simulink model "StemCellStateflow_min"  (R2025b)
settings: Solver=ode4  StartTime=0.0  StopTime=100  FixedStep=0.1  RelTol=1e-3
values from neighbouring files (symbols this model uses):
  RATE_2P = 0.15    [esercizione3_week2.m]
  RATE_2S = 0.30    (= 0.3)    [esercizione3_week2.m]
  RATE_ASYM = 0.50    (= 0.5)    [esercizione3_week2.m]
  RATE_DEATH = 0.05    [esercizione3_week2.m]
  RATE_GRAN = 0.60    (= 0.6)    [esercizione3_week2.m]
  RATE_MACRO = 0.40    (= 0.4)    [esercizione3_week2.m]
settings Model: Creator=aleqs  LastModifiedBy=aleqs

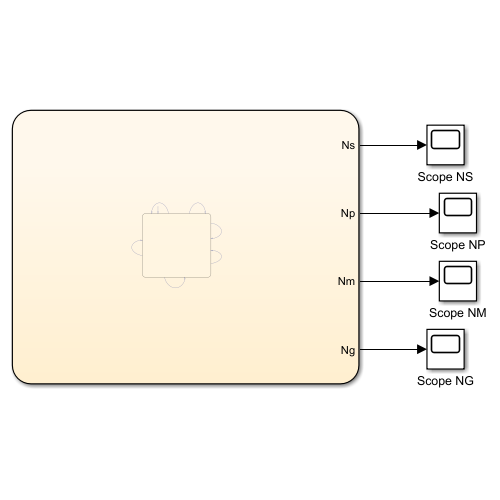
[thumbnail: Simulink's stored preview of the top-level diagram]
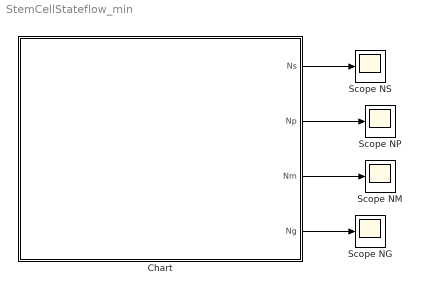
== system StemCellStateflow_min ==
  Chart : Stateflow chart  TreatAsAtomicUnit=on
  Scope NG : Scope
      settings: ActiveDisplayYMinimum=-16.249999999999996  ActiveDisplayYMaximum=146.25  DataLoggingVariableName=ScopeData3
  Scope NM : Scope
      settings: ActiveDisplayYMinimum=-12.630434782608695  ActiveDisplayYMaximum=96.307065217391312  DataLoggingVariableName=ScopeData2
  Scope NP : Scope
      settings: ActiveDisplayYMinimum=35.770917999061176  ActiveDisplayYMaximum=97.75034137796743
  Scope NS : Scope
      settings: ActiveDisplayYMinimum=83.087517832880422  ActiveDisplayYMaximum=137.78529908288044
  wires:
  Chart/4(Ng) -> Scope NG/1
  Chart/3(Nm) -> Scope NM/1
  Chart/2(Np) -> Scope NP/1
  Chart/1(Ns) -> Scope NS/1

== stateflow chart StemCellStateflow_min/Chart ==
  settings: updateMethod=DISCRETE  sampleTime=0.1
  state StemModel
    entry:
    % inizializza orologio
    t = 0;
    % estrai tempi esponenziali per STEM (rate * Ns)
    tau_2S    = -log(rand()) / (RATE_2S  * Ns);
    tau_ASYM  = -log(rand()) / (RATE_ASYM  * Ns);
    tau_2P    = -log(rand()) / (RATE_2P  * Ns);
    tau_DEATH = -log(rand()) / (RATE_DEATH * Ns);
    % estrai tempi per PROGENITORI (se >0)
    if Np > 0
    tau_MACRO = -log(rand()) / (RATE_MACRO * Np);
    tau_GRAN  = -log(rand()) / (RATE_GRAN  * Np);
    else
    tau_MACRO = inf;
    tau_GRAN  = inf;
    end
    during:
    % integra il tempo con passo fisso
    t = t + 0.1;
  StemModel -> StemModel [order 5] : [t >= tau_MACRO && ...
      |  tau_MACRO <= tau_GRAN && tau_MACRO <= tau_2S && ...
      |  tau_MACRO <= tau_ASYM && tau_MACRO <= tau_2P && ...
      |  tau_MACRO <= tau_DEATH && Np > 0]
      | {
      |     Np = Np - 1;
      |     Nm = Nm + 1;
      |     t = 0;
      | }
  StemModel -> StemModel [order 4] : [t >= tau_DEATH && ...
      |  tau_DEATH <= tau_2S && tau_DEATH <= tau_ASYM && tau_DEATH <= tau_2P && ...
      |  tau_DEATH <= tau_MACRO && tau_DEATH <= tau_GRAN && Ns > 0]
      | {
      |     Ns = Ns - 1;
      |     t = 0;
      | }
  (default) -> StemModel
  StemModel -> StemModel [order 6] : [t >= tau_GRAN && tau_GRAN <= tau_MACRO && ...
      |  tau_GRAN <= tau_2S && tau_GRAN <= tau_ASYM && tau_GRAN <= tau_2P && ...
      | tau_GRAN <= tau_DEATH && Np > 0]
      | {
      |     Np = Np - 1;
      |     Ng = Ng + 1;
      |     t = 0;
      | }
  StemModel -> StemModel [order 3] : [t >= tau_2P && ...
      |  tau_2P <= tau_2S && tau_2P <= tau_ASYM && tau_2P <= tau_DEATH && ...
      |  tau_2P <= tau_MACRO && tau_2P <= tau_GRAN && Ns > 0]
      | {
      |     Ns = Ns - 1;
      |     Np = Np + 2;
      |     t = 0;
      | }
  StemModel -> StemModel [order 1] : [t >= tau_2S && ...
      |  tau_2S <= tau_ASYM && tau_2S <= tau_2P && tau_2S <= tau_DEATH && ...
      |  tau_2S <= tau_MACRO && tau_2S <= tau_GRAN && Ns > 0]
      | {
      |     Ns = Ns + 1;
      |     t = 0;
      | }
  StemModel -> StemModel [order 2] : [t >= tau_ASYM && ...
      |  tau_ASYM <= tau_2S && tau_ASYM <= tau_2P && tau_ASYM <= tau_DEATH && ...
      |  tau_ASYM <= tau_MACRO && tau_ASYM <= tau_GRAN && Ns > 0]
      | {
      |     Np = Np + 1;
      |     t = 0;
      | }
  data: Ns output =INITIAL_STEM; t local =0; tau_2S local; tau_ASYM local; Np output =INITIAL_PROG; tau_2P local; tau_DEATH local; Nm output =0; Ng output =0; tau_MACRO local; tau_GRAN local; RATE_2S parameter; RATE_2P parameter; RATE_GRAN parameter; RATE_ASYM parameter; RATE_MACRO parameter; RATE_DEATH parameter
